simulink model "untitled"  (R2022b)
settings: Solver=VariableStepAuto  StartTime=0.0  StopTime=0.1  RelTol=1e-3
values from neighbouring files (symbols this model uses):
  C = Cboost    [hasancan.m]    (also in proje1.m)
  D1 = 1 * 99.99    (= 99.99)    [hasancan.m]    (also in proje1.m; untitled.m)
  D2 = 0.00000001    (= 1e-08)    [hasancan.m]    (also in proje1.m; untitled.m)
  D2_d = 0.00000001    (= 1e-08)    [hasancan.m]    (also in proje1.m; untitled.m)
  D3 = (1 - Dboost) * 99.99    (= 9.89484375)    [hasancan.m]    (also in proje1.m; untitled.m = 36.5348076923)
  D3_d = T * Dboost    (= 1.80208333333e-06)    [hasancan.m]    (also in proje1.m = 3.00347222222e-06; untitled.m = 2.11538461538e-06)
  D4 = Dboost * 99.99    (= 90.09515625)    [hasancan.m]    (also in proje1.m; untitled.m = 63.4551923077)
  L = Lboost    [hasancan.m]    (also in proje1.m)
  R = Po / Io    [hasancan.m]    (also in proje1.m = Po/Io; untitled.m = 13)
  T = 1 / fsw    (= 2e-06)    [hasancan.m]    (also in proje1.m = 3.33333333333e-06; untitled.m = 3.33333333333e-06)
  Vin = round(Vinmin + (Vinmax - Vinmin) * rand(1, 1))    [hasancan.m]    (also in proje1.m = round(Vinmin+(Vinmax-Vinmin)*rand(1,1)); untitled.m)
libraries: spsMosfetLib x4, spsSeriesRLCBranchLib x3, spsCurrentMeasurementLib x1, spsDCVoltageSourceLib x1, spsVoltageMeasurementLib x1, sps_lib x1
settings Model: Creator=hsncn  LastModifiedBy=hsncn

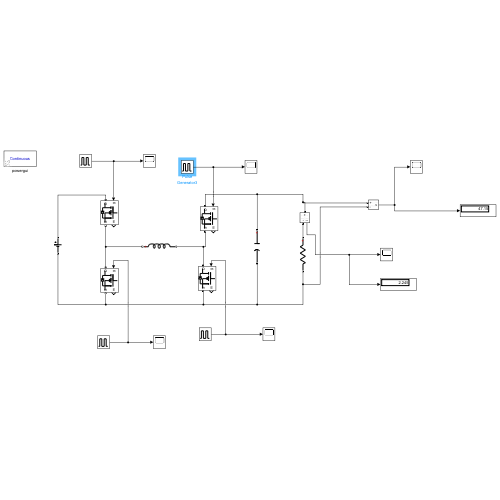
[thumbnail: Simulink's stored preview of the top-level diagram]
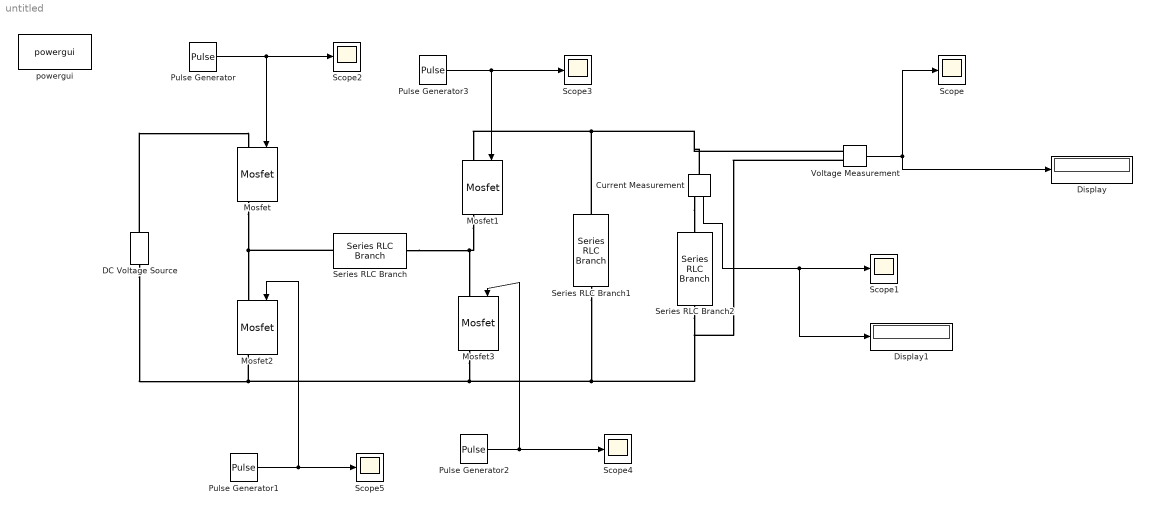
== system untitled ==
  Current Measurement : spsCurrentMeasurementLib/Current Measurement  PhasorSimulation=off  OutputType=Complex  PSBequivalent=0
  DC Voltage Source : spsDCVoltageSourceLib/DC Voltage Source  Amplitude=Vin  Measurements=None
  Display : Display
  Display1 : Display
  Mosfet{,1..3} (4 alike) : spsMosfetLib/Mosfet  Ron=0.1  Lon=0  Rd=0.01  Vfd=0  IC=0  Rs=1e5  Cs=inf  Measurements=on
  Pulse Generator : DiscretePulseGenerator  PulseType=Time based  Period=T  PulseWidth=D1
  Pulse Generator1 : DiscretePulseGenerator  PulseType=Time based  Period=T  PulseWidth=D2  PhaseDelay=D2_d
  Pulse Generator2 : DiscretePulseGenerator  PulseType=Time based  Period=T  PulseWidth=D4
  Pulse Generator3 : DiscretePulseGenerator  PulseType=Time based  Period=T  PulseWidth=D3  PhaseDelay=D3_d
  Scope{,1..5} (6 alike) : Scope
  Series RLC Branch : spsSeriesRLCBranchLib/Series RLC Branch  LConnTagsString=__new0  RConnTagsString=__new0  BranchType=L  Resistance=1  Inductance=L  SetiL0=off  InitialCurrent=0  Capacitance=1e-6  Setx0=off  InitialVoltage=0  Measurements=None
  Series RLC Branch1 : spsSeriesRLCBranchLib/Series RLC Branch  LConnTagsString=__new0  RConnTagsString=__new0  BranchType=C  Resistance=1  Inductance=1e-3  SetiL0=off  InitialCurrent=0  Capacitance=C  Setx0=off  InitialVoltage=0  Measurements=None
  Series RLC Branch2 : spsSeriesRLCBranchLib/Series RLC Branch  LConnTagsString=__new0  RConnTagsString=__new0  BranchType=R  Resistance=R  Inductance=1e-3  SetiL0=off  InitialCurrent=0  Capacitance=1e-6  Setx0=off  InitialVoltage=0  Measurements=None
  Voltage Measurement : spsVoltageMeasurementLib/Voltage Measurement  PhasorSimulation=off  OutputType=Complex  PSBequivalent=0
  powergui : sps_lib/powergui  Priority=1  SimulationMode=Continuous  SampleTime=50e-6  frequency=60  Iterations=50  frequencyindice=0  Pbase=100e6  ErrMax=1e-4  UnitsV=kV  UnitsW=MW  buscounter=0  FunctionMessages=off  echomessages=off  EnableUseOfTLC=off  CurrentSourceSwitches=off  DisableSnubberDevices=off  DisableRonSwitches=off  DisableVfSwitches=off  DisplayEquations=off  AutomaticDiscreteSolvers=off  SolverType=Tustin/Backward Euler (TBE)  Interpol=off  ExternalGateDelay=off  methode=off  Ts=100  x0status=blocks  SPID=on  SwTol=0  HookPort=off  NonlinearTolerance=1e-4  nMaxIteration=100  ContinueOnMaxIteration=off  RestoreLinks=warning  ResistiveCurrentMeasurement=off  Frange=[0:2:500]  Ylog=off  Xlog=on  ShowGrid=off  save=off  variable=ZData  structure=0  ZoomFFT=off  StartTime=0.0  cycles=1  DisplayStyle=1  fundamental=60  FreqAxis=off  MaxFrequency=1000  frequencyindicesteady=1  RmsSteady=1  display=off
  wires:
  Pulse Generator/1 -> Mosfet/1, Scope2/1
  Pulse Generator3/1 -> Mosfet1/1, Scope3/1
  Pulse Generator2/1 -> Scope4/1, Mosfet3/1
  Pulse Generator1/1 -> Mosfet2/1, Scope5/1
  Voltage Measurement/1 -> Scope/1, Display/1
  Current Measurement/1 -> Display1/1, Scope1/1
  connections:
  DC Voltage Source/RConn1 -- Mosfet/LConn1
  DC Voltage Source/LConn1 -- Voltage Measurement/LConn2 -- Series RLC Branch2/RConn1 -- Series RLC Branch1/RConn1 -- Mosfet3/RConn1 -- Mosfet2/RConn1
  Mosfet/RConn1 -- Mosfet2/LConn1 -- Series RLC Branch/LConn1
  Mosfet1/RConn1 -- Series RLC Branch/RConn1 -- Mosfet3/LConn1
  Series RLC Branch1/LConn1 -- Current Measurement/LConn1 -- Voltage Measurement/LConn1 -- Mosfet1/LConn1
  Current Measurement/RConn1 -- Series RLC Branch2/LConn1
